simulink model "TempCorrect_OfflineTest_Automated"  (R2014a)
settings: Solver=ode3  StartTime=0.0  StopTime=Gyro.time(end)  FixedStep=1/400  RelTol=1e-3
PostLoadFcn:
  | Gyro_Correction_Roll.P1  = 0;
  | Gyro_Correction_Roll.P2 = 1;
  | Gyro_Correction_Roll.Offset = 0;
  | 
  | Gyro_Correction_Pitch.P1  = 0;
  | Gyro_Correction_Pitch.P2 = 1;
  | Gyro_Correction_Pitch.Offset = 0;
  | 
  | Gyro_Correction_Yaw.P1  = 0;
  | Gyro_Correction_Yaw.P2 = 1;
  | Gyro_Correction_Yaw.Offset = 0;
undefined symbols (not defined in the file or in its folder): DiscIntNeverNeededParam
settings Model: ExtModeTrigDuration=40001  Creator=darenlee  LastModifiedBy=darenlee
settings DataIOCC: SignalLoggingSaveFormat=ModelDataLogs
settings DebuggingCC: MultiTaskDSMMsg=warning  MultiTaskCondExecSysMsg=none
settings RTWCC: IncludeERTFirstTime=on

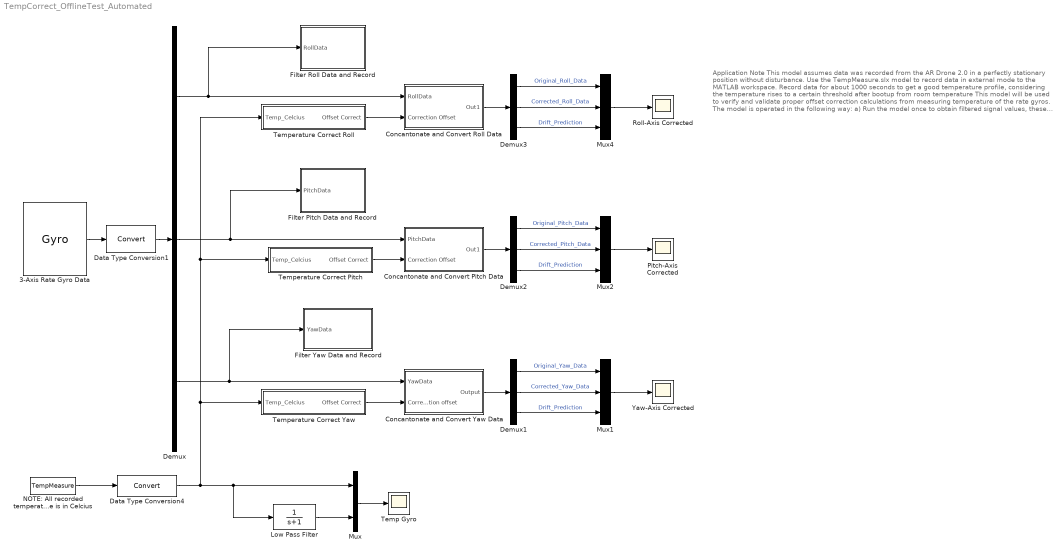
== system TempCorrect_OfflineTest_Automated ==
  note: Application Note
      |
      | This model assumes data was recorded from the AR Drone 2.0 in a perfectly stationary position without disturbance. Use the TempMeasure.slx model to record data in external mode to the MATLAB workspace. Record data for about 1000 seconds to get a good temperature profile, considering the temperature rises to a certain threshold after bootup from room temperature
      |
      | This model will be used to verify and validate proper
      | offset correction calculations from measuring temperature of the rate gyros. The model is operated
      | in the following way:
      |
      | a)
      | Run the model once to obtain filtered signal values, these filtered signals are primarily of temperature and the rate gyros. Since these signals are rather noisy we want to be able to find the average value of these signals to get a better estimate of the offset parameters
      |
      | b)
      | Run the script 'Temperature_Testing_Automated_Script.m'. This will perform an automated curve fitting routine
      | 'TempMeasureRefined' which is the indepdent 'x' variable
      | 'GyroDrift_Roll' which is the dependent 'y' variable
      |
      | and so forth
      |
      | The parameters inside these subsystems are updated with the appropiate gain and offset corrections
      | \Temperature Correct Roll
      | \Temperature Correct Pitch
      | \Temperature Correct Yaw
      |
      | NOTE:
      | It may be advantageous to have a third term in the polynomial (x^2 term) if it gives a slightly better fit. update the structure appropiately for the p1 term. The script will auto-populate the p2 and p3 term being gain and offset, but p1 was set to zero for no quadratic term
      |
      | c)
      | Now, we'r eready to validate. Press the play button and look at the scopes.
      | Yellow Signal - The original uncorrected data not centered at zero
      | Purple Signal - Corrected data. This should be centered at zero
      | Teal Signal - The purpose of this is to examine integration drift.. it is a measurement of how effective our correction factor removed the drift bias. If one were to integrate the purple signal, ideally the reported attitude should be zero or close to it. Minor drift is acceptable since the AHRS system will take care of the rest
  3-Axis Rate Gyro Data : FromWorkspace  VariableName=Gyro
  Concantonate and Convert Pitch Data : Subsystem
  Concantonate and Convert Roll Data : Subsystem
  Concantonate and Convert Yaw Data : Subsystem
  Data Type Conversion1 : DataTypeConversion
  Data Type Conversion4 : DataTypeConversion
  Demux{,1..3} (4 alike) : Demux  Outputs=3
  Filter Pitch Data and Record : Subsystem
  Filter Roll Data and Record : Subsystem
  Filter Yaw Data and Record : Subsystem
  Low Pass Filter : TransferFcn  Denominator=[1 1]
  Mux : Mux  Inputs=2
  Mux1 : Mux  Inputs=3
  Mux2 : Mux  Inputs=3
  Mux4 : Mux  Inputs=3
  NOTE: All recorded temperature is in Celcius : FromWorkspace  VariableName=TempMeasure
  Pitch-Axis Corrected : Scope
      settings: ShowLegends=on  YMax=37.5  SaveName=Pitch_Corrected_Uncorrected
  Roll-Axis Corrected : Scope
      settings: ShowLegends=on  TimeRange=571.1351351351351  YMin=-10  YMax=120  SaveName=ForDocumentation
  Temp Gyro : Scope
      settings: YMin=46  YMax=48.75  SaveName=FilteredTemp
  Temperature Correct Pitch : Subsystem
  Temperature Correct Roll : Subsystem
  Temperature Correct Yaw : Subsystem
  Yaw-Axis Corrected : Scope
      settings: ShowLegends=on  YMin=-7  YMax=4  SaveName=Roll_Corrected_Uncorrected2
  wires:
  3-Axis Rate Gyro Data/1 -> Data Type Conversion1/1
  NOTE: All recorded temperature is in Celcius/1 -> Data Type Conversion4/1
  Data Type Conversion1/1 -> Demux/1
  Demux/1 -> Concantonate and Convert Roll Data/1(RollData), Filter Roll Data and Record/1(RollData)
  Data Type Conversion4/1 -> Mux/1, Low Pass Filter/1, Temperature Correct Yaw/1(Temp_Celcius), Temperature Correct Pitch/1(Temp_Celcius), Temperature Correct Roll/1(Temp_Celcius)
  Mux/1 -> Temp Gyro/1
  Demux/3 -> Concantonate and Convert Yaw Data/1(YawData), Filter Yaw Data and Record/1(YawData)
  Low Pass Filter/1 -> Mux/2
  Demux/2 -> Concantonate and Convert Pitch Data/1(PitchData), Filter Pitch Data and Record/1(PitchData)
  Temperature Correct Yaw/1(Offset Correct) -> Concantonate and Convert Yaw Data/2(Correction offset)
  Concantonate and Convert Yaw Data/1(Output) -> Demux1/1
  Demux1/1 -> Mux1/1  "Original_Yaw_Data"
  Demux1/2 -> Mux1/2  "Corrected_Yaw_Data"
  Demux1/3 -> Mux1/3  "Drift_Prediction"
  Mux1/1 -> Yaw-Axis Corrected/1
  Temperature Correct Pitch/1(Offset Correct) -> Concantonate and Convert Pitch Data/2(Correction Offset)
  Concantonate and Convert Pitch Data/1(Out1) -> Demux2/1
  Demux2/1 -> Mux2/1  "Original_Pitch_Data"
  Demux2/2 -> Mux2/2  "Corrected_Pitch_Data"
  Demux2/3 -> Mux2/3  "Drift_Prediction"
  Mux2/1 -> Pitch-Axis Corrected/1
  Demux3/1 -> Mux4/1  "Original_Roll_Data"
  Demux3/2 -> Mux4/2  "Corrected_Roll_Data"
  Demux3/3 -> Mux4/3  "Drift_Prediction"
  Concantonate and Convert Roll Data/1(Out1) -> Demux3/1
  Mux4/1 -> Roll-Axis Corrected/1
  Temperature Correct Roll/1(Offset Correct) -> Concantonate and Convert Roll Data/2(Correction Offset)

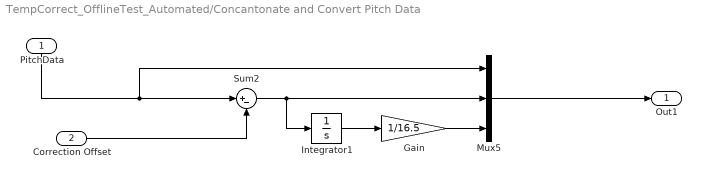
== system TempCorrect_OfflineTest_Automated/Concantonate and Convert Pitch Data ==
  PitchData : Inport
  Correction Offset : Inport  Port=2
  Gain : Gain  Gain=1/16.5
  Integrator1 : Integrator
  Mux5 : Mux  Inputs=3
  Sum2 : Sum  Inputs=|+-
  Out1 : Outport
  wires:
  Mux5/1 -> Out1/1
  Sum2/1 -> Integrator1/1, Mux5/2
  Correction Offset/1 -> Sum2/2
  Gain/1 -> Mux5/3
  Integrator1/1 -> Gain/1
  PitchData/1 -> Mux5/1, Sum2/1

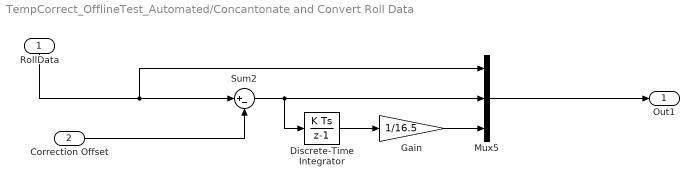
== system TempCorrect_OfflineTest_Automated/Concantonate and Convert Roll Data ==
  RollData : Inport
  Correction Offset : Inport  Port=2
  Discrete-Time Integrator : DiscreteIntegrator  SampleTime=1/400  ICPrevOutput=DiscIntNeverNeededParam  ICPrevScaledInput=DiscIntNeverNeededParam
  Gain : Gain  Gain=1/16.5
  Mux5 : Mux  Inputs=3
  Sum2 : Sum  Inputs=|+-
  Out1 : Outport
  wires:
  Mux5/1 -> Out1/1
  Sum2/1 -> Discrete-Time Integrator/1, Mux5/2
  Correction Offset/1 -> Sum2/2
  Gain/1 -> Mux5/3
  Discrete-Time Integrator/1 -> Gain/1
  RollData/1 -> Mux5/1, Sum2/1

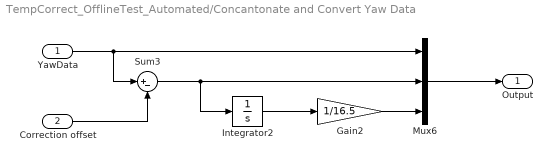
== system TempCorrect_OfflineTest_Automated/Concantonate and Convert Yaw Data ==
  YawData : Inport
  Correction offset : Inport  Port=2
  Gain2 : Gain  Gain=1/16.5
  Integrator2 : Integrator
  Mux6 : Mux  Inputs=3
  Sum3 : Sum  Inputs=|+-
  Output : Outport
  wires:
  Sum3/1 -> Integrator2/1, Mux6/2
  Correction offset/1 -> Sum3/2
  Integrator2/1 -> Gain2/1
  Mux6/1 -> Output/1
  Gain2/1 -> Mux6/3
  YawData/1 -> Sum3/1, Mux6/1

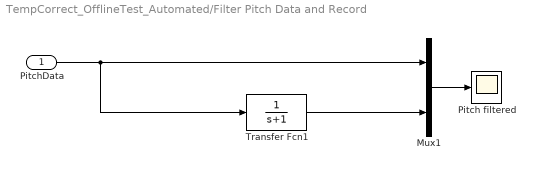
== system TempCorrect_OfflineTest_Automated/Filter Pitch Data and Record ==
  PitchData : Inport
  Mux1 : Mux  Inputs=2
  Pitch filtered : Scope
      settings: SaveName=Pitch_Gyro_filtered
  Transfer Fcn1 : TransferFcn  Denominator=[1 1]
  wires:
  Transfer Fcn1/1 -> Mux1/2
  Mux1/1 -> Pitch filtered/1
  PitchData/1 -> Transfer Fcn1/1, Mux1/1

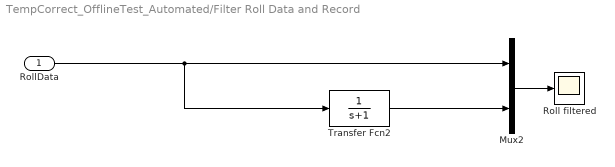
== system TempCorrect_OfflineTest_Automated/Filter Roll Data and Record ==
  RollData : Inport
  Mux2 : Mux  Inputs=2
  Roll filtered : Scope
      settings: SaveName=Roll_Gyro_filtered
  Transfer Fcn2 : TransferFcn  Denominator=[1 1]
  wires:
  Mux2/1 -> Roll filtered/1
  Transfer Fcn2/1 -> Mux2/2
  RollData/1 -> Transfer Fcn2/1, Mux2/1

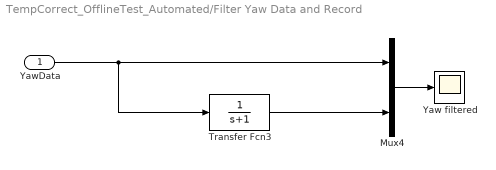
== system TempCorrect_OfflineTest_Automated/Filter Yaw Data and Record ==
  YawData : Inport
  Mux4 : Mux  Inputs=2
  Transfer Fcn3 : TransferFcn  Denominator=[1 1]
  Yaw filtered : Scope
      settings: SaveName=Yaw_Gyro_filtered
  wires:
  Mux4/1 -> Yaw filtered/1
  Transfer Fcn3/1 -> Mux4/2
  YawData/1 -> Transfer Fcn3/1, Mux4/1

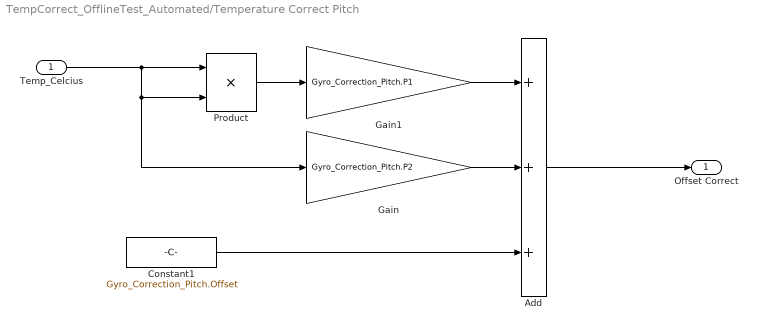
== system TempCorrect_OfflineTest_Automated/Temperature Correct Pitch ==
  Temp_Celcius : Inport
  Add : Sum  Inputs=+++
  Constant1 : Constant  Value=Gyro_Correction_Pitch.Offset
      settings: AttributesFormatString=%<Value>
  Gain : Gain  Gain=Gyro_Correction_Pitch.P2
      settings: AttributesFormatString=%<Gain>
  Gain1 : Gain  Gain=Gyro_Correction_Pitch.P1
      settings: AttributesFormatString=%<Gain>
  Product : Product
  Offset Correct : Outport
  wires:
  Temp_Celcius/1 -> Gain/1, Product/2, Product/1
  Constant1/1 -> Add/3
  Add/1 -> Offset Correct/1
  Product/1 -> Gain1/1
  Gain1/1 -> Add/1
  Gain/1 -> Add/2

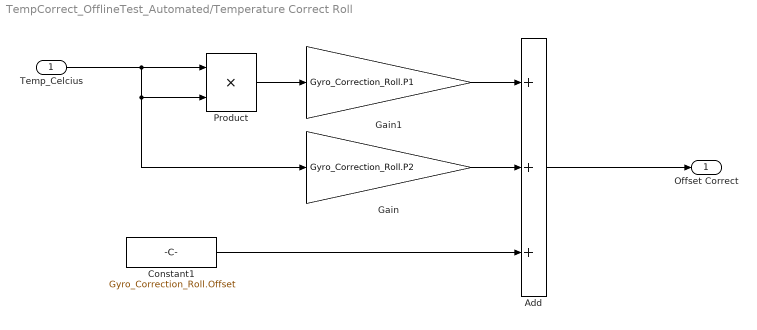
== system TempCorrect_OfflineTest_Automated/Temperature Correct Roll ==
  Temp_Celcius : Inport
  Add : Sum  Inputs=+++
  Constant1 : Constant  Value=Gyro_Correction_Roll.Offset
      settings: AttributesFormatString=%<Value>
  Gain : Gain  Gain=Gyro_Correction_Roll.P2
      settings: AttributesFormatString=%<Gain>
  Gain1 : Gain  Gain=Gyro_Correction_Roll.P1
      settings: AttributesFormatString=%<Gain>
  Product : Product
  Offset Correct : Outport
  wires:
  Temp_Celcius/1 -> Gain/1, Product/2, Product/1
  Constant1/1 -> Add/3
  Add/1 -> Offset Correct/1
  Product/1 -> Gain1/1
  Gain1/1 -> Add/1
  Gain/1 -> Add/2

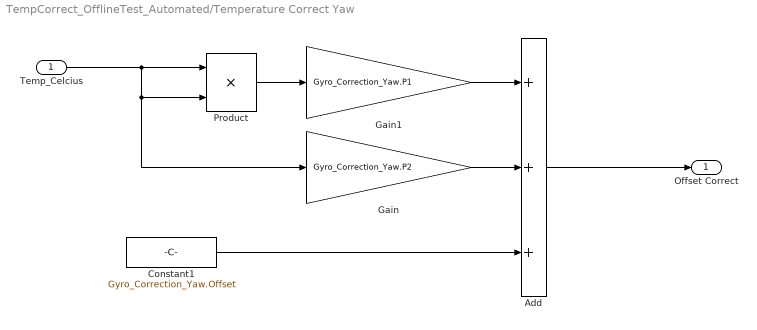
== system TempCorrect_OfflineTest_Automated/Temperature Correct Yaw ==
  Temp_Celcius : Inport
  Add : Sum  Inputs=+++
  Constant1 : Constant  Value=Gyro_Correction_Yaw.Offset
      settings: AttributesFormatString=%<Value>
  Gain : Gain  Gain=Gyro_Correction_Yaw.P2
      settings: AttributesFormatString=%<Gain>
  Gain1 : Gain  Gain=Gyro_Correction_Yaw.P1
      settings: AttributesFormatString=%<Gain>
  Product : Product
  Offset Correct : Outport
  wires:
  Temp_Celcius/1 -> Gain/1, Product/2, Product/1
  Constant1/1 -> Add/3
  Add/1 -> Offset Correct/1
  Product/1 -> Gain1/1
  Gain1/1 -> Add/1
  Gain/1 -> Add/2
